simulink library "NSA_DEVS_DIGITAL_LOGIC"  (R2022b)
settings: Solver=VariableStepAuto  StartTime=0.0  StopTime=10.0  RelTol=1e-3
libraries: $bdroot x8
settings Model: Creator=david  LastModifiedBy=david

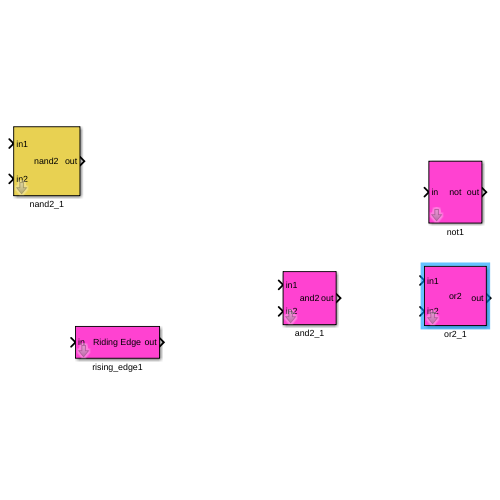
[thumbnail: Simulink's stored preview of the top-level diagram]
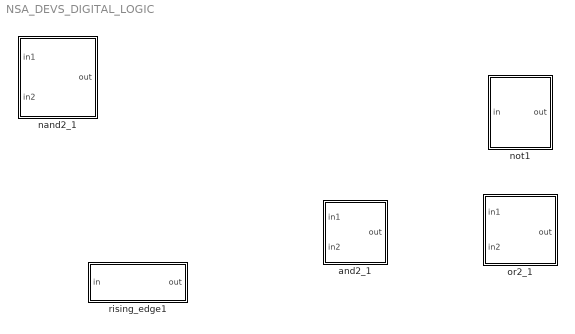
== system NSA_DEVS_DIGITAL_LOGIC ==
  and2_1 : Subsystem  mask{tau=[0,1], debug=0, constructor='and2("name", tau, debug)'}
      mask Display:
      | disp("and2");
      | 
      | port_label('input', 1, 'in1');
      | port_label('input', 2, 'in2');
      | port_label('output', 1, 'out');
  nand2_1 : Subsystem  mask{tau=[0,1], debug=0, constructor='nand2("name", tau, debug)'}
      mask Display:
      | disp("nand2");
      | 
      | port_label('input', 1, 'in1');
      | port_label('input', 2, 'in2');
      | port_label('output', 1, 'out');
  not1 : Subsystem  mask{tau=[0,1], debug=0, constructor='not("name",tau,debug)'}
      mask Display:
      | disp("not");
      | 
      | port_label('input', 1, 'in');
      | port_label('output', 1, 'out');
  or2_1 : Subsystem  mask{tau=[0,1], debug=0, constructor='or2("name", tau, debug)'}
      mask Display:
      | disp("or2");
      | 
      | port_label('input', 1, 'in1');
      | port_label('input', 2, 'in2');
      | port_label('output', 1, 'out');
  rising_edge1 : Subsystem  mask{tau=[0,1], debug=0, constructor='Rising_Edge("name", tau, debug)'}
      mask Display:
      | disp("Riding Edge");
      | 
      | port_label('input', 1, 'in');
      | port_label('output', 1, 'out');

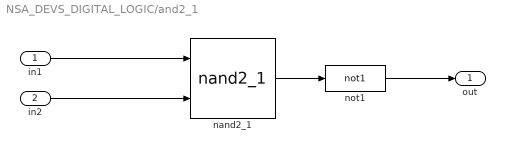
== system NSA_DEVS_DIGITAL_LOGIC/and2_1 ==
  in1 : Inport
  in2 : Inport  Port=2
  nand2_1 : $bdroot/nand2_1  tau=[0,1]  debug=debug  constructor="'nand2(\"name\", tau, debug)'"
      settings: LibrarySourceBlock=NSA_DEVS_LIB/nand2_1
  not1 : $bdroot/not1  tau=tau  debug=debug  constructor="'not(\"name\",tau,debug)'"
      settings: LibrarySourceBlock=NSA_DEVS_LIB/not1
  out : Outport
  wires:
  in2/1 -> nand2_1/2
  not1/1 -> out/1
  nand2_1/1 -> not1/1
  in1/1 -> nand2_1/1

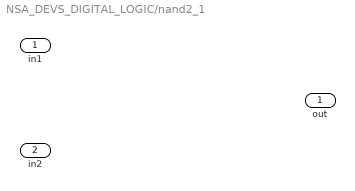
== system NSA_DEVS_DIGITAL_LOGIC/nand2_1 ==
  in1 : Inport
  in2 : Inport  Port=2
  out : Outport

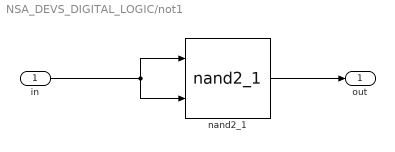
== system NSA_DEVS_DIGITAL_LOGIC/not1 ==
  in : Inport
  nand2_1 : $bdroot/nand2_1  tau=tau  debug=debug  constructor="'nand2(\"name\", tau, debug)'"
      settings: LibrarySourceBlock=NSA_DEVS_LIB/nand2_1
  out : Outport
  wires:
  nand2_1/1 -> out/1
  in/1 -> nand2_1/1, nand2_1/2

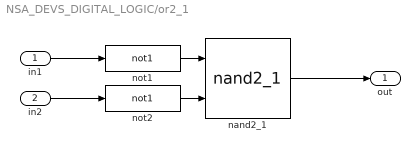
== system NSA_DEVS_DIGITAL_LOGIC/or2_1 ==
  in1 : Inport
  in2 : Inport  Port=2
  nand2_1 : $bdroot/nand2_1  tau=[0,1]  debug=debug  constructor="'nand2(\"name\", tau, debug)'"
      settings: LibrarySourceBlock=NSA_DEVS_LIB/nand2_1
  not1 : $bdroot/not1  tau=tau  debug=debug  constructor="'not(\"name\",tau,debug)'"
      settings: LibrarySourceBlock=NSA_DEVS_LIB/not1
  not2 : $bdroot/not1  tau=tau  debug=debug  constructor="'not(\"name\",tau,debug)'"
      settings: LibrarySourceBlock=NSA_DEVS_LIB/not1
  out : Outport
  wires:
  not1/1 -> nand2_1/1
  not2/1 -> nand2_1/2
  in2/1 -> not2/1
  in1/1 -> not1/1
  nand2_1/1 -> out/1

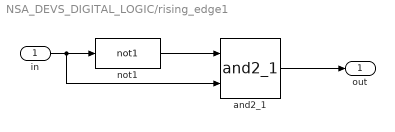
== system NSA_DEVS_DIGITAL_LOGIC/rising_edge1 ==
  in : Inport
  and2_1 : $bdroot/and2_1  tau=tau  debug=debug  constructor="'and2(\"name\", tau, debug)'"
      settings: LibrarySourceBlock=NSA_DEVS_LIB/and2_1
  not1 : $bdroot/not1  tau=2*tau  debug=debug  constructor="'not(\"name\",tau,debug)'"
      settings: LibrarySourceBlock=NSA_DEVS_LIB/not1
  out : Outport
  wires:
  in/1 -> and2_1/2, not1/1
  not1/1 -> and2_1/1
  and2_1/1 -> out/1
